simulink model "ModeStEnCtrl6s7sPreCondition"  (R2018b)
settings: Solver=FixedStepDiscrete  StartTime=0.0  StopTime=10.0  RelTol=1e-3
undefined symbols (not defined in the file or in its folder): KeSMSuSecRwStBackPosDelta_Val
libraries: simulink x2
settings Model: Creator=sn2xws  LastModifiedBy=sn2xws
settings DataIOCC: SaveFormat=StructureWithTime
settings OptimizationCC: DefaultParameterBehavior=Inlined  EnhancedBackFolding=on  PassReuseOutputArgsAs=Individual arguments  ZeroExternalMemoryAtStartup=off  ZeroInternalMemoryAtStartup=off  OptimizeBlockOrder=speed  DifferentSizesBufferReuse=on  OptimizationCustomize=off
settings DebuggingCC: ParameterTunabilityLossMsg=error
settings SFSimCC: MATLABDynamicMemAlloc=off
settings RTWCC: SystemTargetFile=autosar.tlc  GenCodeOnly=on  TemplateMakefile=ert_default_tmf  Description=AUTOSAR  GenerateReport=on  IncludeHyperlinkInReport=on  LaunchReport=on  GenerateTraceInfo=on  GenerateTraceReport=on  GenerateTraceReportSl=on  GenerateTraceReportSf=on  GenerateTraceReportEml=on  GenerateCodeMetricsReport=on
settings CodeAppCC: ForceParamTrailComments=on  IgnoreCustomStorageClasses=off  OperatorAnnotations=on  SimulinkDataObjDesc=on  SFDataObjDesc=on  InsertBlockDesc=on
settings STFCustomTargetCC: TargetLangStandard=C99 (ISO)  MultiwordLength=256  ParMdlRefBuildCompliant=on  CompOptLevelCompliant=on  IncludeMdlTerminateFcn=off  CombineOutputUpdateFcns=on  SuppressErrorStatus=on  ERTCustomFileBanners=on  SupportNonFinite=off  SupportComplex=off  SupportContinuousTime=off  SupportNonInlinedSFcns=off  RemoveResetFunc=on  MATLABClassNameForMDSCustomization=Simulink.SoftwareTarget.ERTCustomization  AutosarCompliant=on  UseToolchainInfoCompliant=on  LookupTableObjectStructAxisOrder=2,1,3,4,...  LUTObjectStructOrderEvenSpacing=Size,Table,Breakpoints  SystemTargetFile=autosar.tlc
settings ERTTargetCC: TargetLangStandard=C99 (ISO)  ConcurrentExecutionCompliant=off  IncludeMdlTerminateFcn=off  SuppressErrorStatus=on  SupportNonFinite=off  SupportComplex=off  ModelStepFunctionPrototypeControlCompliant=off  CPPClassGenCompliant=off  AutosarCompliant=on  LookupTableObjectStructAxisOrder=2,1,3,4,...  LUTObjectStructOrderEvenSpacing=Size,Table,Breakpoints  InlinedParameterPlacement=NonHierarchical  ERTCustomFileTemplate=example_file_process.tlc  ERTFilePackagingFormat=Compact

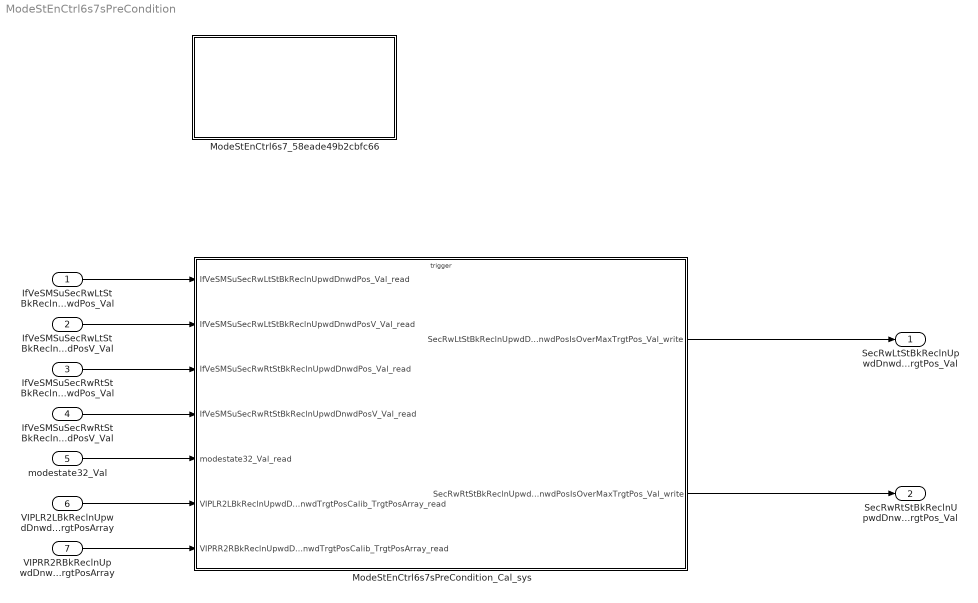
== system ModeStEnCtrl6s7sPreCondition ==
  IfVeSMSuSecRwLtStBkReclnUpwdDnwdPos_Val : Inport  OutDataTypeStr=uint16  PortDimensions=1
  IfVeSMSuSecRwLtStBkReclnUpwdDnwdPosV_Val : Inport  Port=2  OutDataTypeStr=boolean  PortDimensions=1
  IfVeSMSuSecRwRtStBkReclnUpwdDnwdPos_Val : Inport  Port=3  OutDataTypeStr=uint16  PortDimensions=1
  IfVeSMSuSecRwRtStBkReclnUpwdDnwdPosV_Val : Inport  Port=4  OutDataTypeStr=boolean  PortDimensions=1
  modestate32_Val : Inport  Port=5  OutDataTypeStr=uint32  PortDimensions=1
  VIPLR2LBkReclnUpwdDnwdTrgtPosCalib_TrgtPosArray : Inport  Description=|  Port=6  OutDataTypeStr=uint16  PortDimensions=3
      | 0:Pos
      | 1:Max
      | 2:Min
  VIPRR2RBkReclnUpwdDnwdTrgtPosCalib_TrgtPosArray : Inport  Description=|  Port=7  OutDataTypeStr=uint16  PortDimensions=3
      | 0:Pos
      | 1:Max
      | 2:Min
  ModeStEnCtrl6s7_58eade49b2cbfc66 : Subsystem
  ModeStEnCtrl6s7sPreCondition_Cal_sys : Subsystem
  SecRwLtStBkReclnUpwdDnwdPosIsOverMaxTrgtPos_Val : Outport  OutDataTypeStr=boolean  PortDimensions=1
  SecRwRtStBkReclnUpwdDnwdPosIsOverMaxTrgtPos_Val : Outport  Port=2  OutDataTypeStr=boolean  PortDimensions=1
  wires:
  IfVeSMSuSecRwLtStBkReclnUpwdDnwdPos_Val/1 -> ModeStEnCtrl6s7sPreCondition_Cal_sys/1(IfVeSMSuSecRwLtStBkReclnUpwdDnwdPos_Val_read)
  IfVeSMSuSecRwLtStBkReclnUpwdDnwdPosV_Val/1 -> ModeStEnCtrl6s7sPreCondition_Cal_sys/2(IfVeSMSuSecRwLtStBkReclnUpwdDnwdPosV_Val_read)
  IfVeSMSuSecRwRtStBkReclnUpwdDnwdPos_Val/1 -> ModeStEnCtrl6s7sPreCondition_Cal_sys/3(IfVeSMSuSecRwRtStBkReclnUpwdDnwdPos_Val_read)
  IfVeSMSuSecRwRtStBkReclnUpwdDnwdPosV_Val/1 -> ModeStEnCtrl6s7sPreCondition_Cal_sys/4(IfVeSMSuSecRwRtStBkReclnUpwdDnwdPosV_Val_read)
  modestate32_Val/1 -> ModeStEnCtrl6s7sPreCondition_Cal_sys/5(modestate32_Val_read)
  VIPLR2LBkReclnUpwdDnwdTrgtPosCalib_TrgtPosArray/1 -> ModeStEnCtrl6s7sPreCondition_Cal_sys/6(VIPLR2LBkReclnUpwdDnwdTrgtPosCalib_TrgtPosArray_read)
  VIPRR2RBkReclnUpwdDnwdTrgtPosCalib_TrgtPosArray/1 -> ModeStEnCtrl6s7sPreCondition_Cal_sys/7(VIPRR2RBkReclnUpwdDnwdTrgtPosCalib_TrgtPosArray_read)
  ModeStEnCtrl6s7sPreCondition_Cal_sys/1(SecRwLtStBkReclnUpwdDnwdPosIsOverMaxTrgtPos_Val_write) -> SecRwLtStBkReclnUpwdDnwdPosIsOverMaxTrgtPos_Val/1
  ModeStEnCtrl6s7sPreCondition_Cal_sys/2(SecRwRtStBkReclnUpwdDnwdPosIsOverMaxTrgtPos_Val_write) -> SecRwRtStBkReclnUpwdDnwdPosIsOverMaxTrgtPos_Val/1

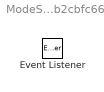
== system ModeStEnCtrl6s7sPreCondition/ModeStEnCtrl6s7_58eade49b2cbfc66 ==
  Event Listener : EventListener  EventName=reset

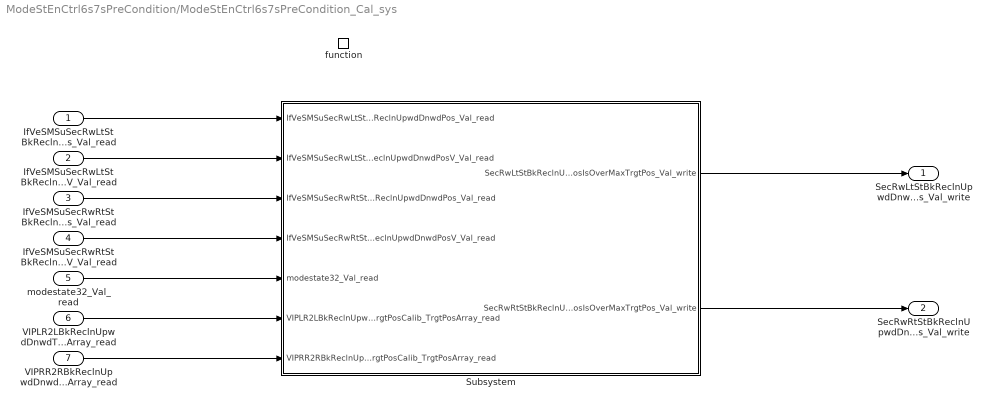
== system ModeStEnCtrl6s7sPreCondition/ModeStEnCtrl6s7sPreCondition_Cal_sys ==
  IfVeSMSuSecRwLtStBkReclnUpwdDnwdPos_Val_read : Inport
  IfVeSMSuSecRwLtStBkReclnUpwdDnwdPosV_Val_read : Inport  Port=2
  IfVeSMSuSecRwRtStBkReclnUpwdDnwdPos_Val_read : Inport  Port=3
  IfVeSMSuSecRwRtStBkReclnUpwdDnwdPosV_Val_read : Inport  Port=4
  modestate32_Val_read : Inport  Port=5
  VIPLR2LBkReclnUpwdDnwdTrgtPosCalib_TrgtPosArray_read : Inport  Port=6
  VIPRR2RBkReclnUpwdDnwdTrgtPosCalib_TrgtPosArray_read : Inport  Port=7
  function : TriggerPort  TriggerType=function-call  IsSimulinkFunction=on  FunctionName=ModeStEnCtrl6s7sPreCondition_Cal  VariantControl=(inherit)
  Subsystem : Subsystem
  SecRwLtStBkReclnUpwdDnwdPosIsOverMaxTrgtPos_Val_write : Outport
      settings: EnsureOutportIsVirtual=on
  SecRwRtStBkReclnUpwdDnwdPosIsOverMaxTrgtPos_Val_write : Outport  Port=2
      settings: EnsureOutportIsVirtual=on
  wires:
  IfVeSMSuSecRwLtStBkReclnUpwdDnwdPos_Val_read/1 -> Subsystem/1(IfVeSMSuSecRwLtStBkReclnUpwdDnwdPos_Val_read)
  IfVeSMSuSecRwLtStBkReclnUpwdDnwdPosV_Val_read/1 -> Subsystem/2(IfVeSMSuSecRwLtStBkReclnUpwdDnwdPosV_Val_read)
  IfVeSMSuSecRwRtStBkReclnUpwdDnwdPos_Val_read/1 -> Subsystem/3(IfVeSMSuSecRwRtStBkReclnUpwdDnwdPos_Val_read)
  IfVeSMSuSecRwRtStBkReclnUpwdDnwdPosV_Val_read/1 -> Subsystem/4(IfVeSMSuSecRwRtStBkReclnUpwdDnwdPosV_Val_read)
  modestate32_Val_read/1 -> Subsystem/5(modestate32_Val_read)
  VIPLR2LBkReclnUpwdDnwdTrgtPosCalib_TrgtPosArray_read/1 -> Subsystem/6(VIPLR2LBkReclnUpwdDnwdTrgtPosCalib_TrgtPosArray_read)
  VIPRR2RBkReclnUpwdDnwdTrgtPosCalib_TrgtPosArray_read/1 -> Subsystem/7(VIPRR2RBkReclnUpwdDnwdTrgtPosCalib_TrgtPosArray_read)
  Subsystem/1(SecRwLtStBkReclnUpwdDnwdPosIsOverMaxTrgtPos_Val_write) -> SecRwLtStBkReclnUpwdDnwdPosIsOverMaxTrgtPos_Val_write/1
  Subsystem/2(SecRwRtStBkReclnUpwdDnwdPosIsOverMaxTrgtPos_Val_write) -> SecRwRtStBkReclnUpwdDnwdPosIsOverMaxTrgtPos_Val_write/1

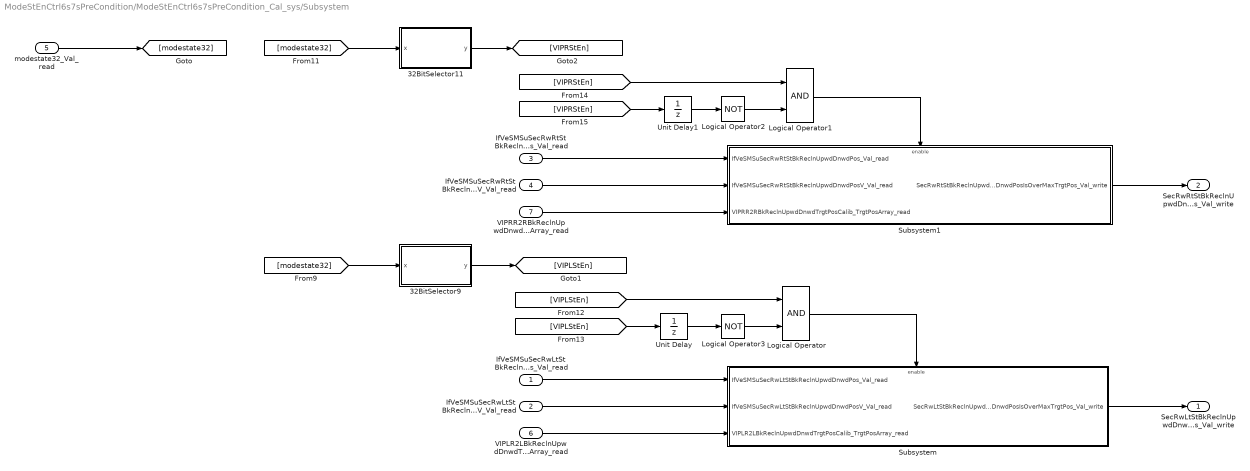
== system ModeStEnCtrl6s7sPreCondition/ModeStEnCtrl6s7sPreCondition_Cal_sys/Subsystem ==
  IfVeSMSuSecRwLtStBkReclnUpwdDnwdPos_Val_read : Inport
  IfVeSMSuSecRwLtStBkReclnUpwdDnwdPosV_Val_read : Inport  Port=2
  IfVeSMSuSecRwRtStBkReclnUpwdDnwdPos_Val_read : Inport  Port=3
  IfVeSMSuSecRwRtStBkReclnUpwdDnwdPosV_Val_read : Inport  Port=4
  modestate32_Val_read : Inport  Port=5
  VIPLR2LBkReclnUpwdDnwdTrgtPosCalib_TrgtPosArray_read : Inport  Port=6
  VIPRR2RBkReclnUpwdDnwdTrgtPosCalib_TrgtPosArray_read : Inport  Port=7
  32BitSelector11 : Subsystem  mask(32 Bit Selector){BitNum=11}
      mask prompts: BitNum "Select Bit Number"
      mask help: Allows selection of a particular bit (0-31) out of a packed word up to 32 bits long. Output will be true if the bit number selected via the mask parameter is equal to one.
      mask TypeOptions BitNum: 0 | 1 | 2 | 3 | 4 | 5 | 6 | 7 | 8 | 9 | 10 | 11 | 12 | 13 | 14 | 15 | 16 | 17 | 18 | 19 | 20 | 21 | 22 | 23 | 24 | 25 | 26 | 27 | 28 | 29 | 30 | 31
      mask Display:
      | text(0.5, 0.8,'BIT','horizontalAlignment','center')
      | text(0.5, 0.5,'SELECTOR','horizontalAlignment','center')
      | text(0.5, 0.2,['-- Bit ',char(get_param(gcb,'BitNum')),' --'],'horizontalAlignment','center')
  32BitSelector9 : Subsystem  mask(32 Bit Selector){BitNum=9}
      mask prompts: BitNum "Select Bit Number"
      mask help: Allows selection of a particular bit (0-31) out of a packed word up to 32 bits long. Output will be true if the bit number selected via the mask parameter is equal to one.
      mask TypeOptions BitNum: 0 | 1 | 2 | 3 | 4 | 5 | 6 | 7 | 8 | 9 | 10 | 11 | 12 | 13 | 14 | 15 | 16 | 17 | 18 | 19 | 20 | 21 | 22 | 23 | 24 | 25 | 26 | 27 | 28 | 29 | 30 | 31
      mask Display:
      | text(0.5, 0.8,'BIT','horizontalAlignment','center')
      | text(0.5, 0.5,'SELECTOR','horizontalAlignment','center')
      | text(0.5, 0.2,['-- Bit ',char(get_param(gcb,'BitNum')),' --'],'horizontalAlignment','center')
  Logical Operator : Logic  AllPortsSameDT=off  OutDataTypeStr=boolean
  Logical Operator1 : Logic  AllPortsSameDT=off  OutDataTypeStr=boolean
  Logical Operator2 : Logic  Operator=NOT  AllPortsSameDT=off  OutDataTypeStr=boolean
  Logical Operator3 : Logic  Operator=NOT  AllPortsSameDT=off  OutDataTypeStr=boolean
  Subsystem : Subsystem
  Subsystem1 : Subsystem
  Unit Delay : UnitDelay  SampleTime=-1
  Unit Delay1 : UnitDelay  SampleTime=-1
  SecRwLtStBkReclnUpwdDnwdPosIsOverMaxTrgtPos_Val_write : Outport
      settings: EnsureOutportIsVirtual=on
  SecRwRtStBkReclnUpwdDnwdPosIsOverMaxTrgtPos_Val_write : Outport  Port=2
      settings: EnsureOutportIsVirtual=on
  wires:
  IfVeSMSuSecRwRtStBkReclnUpwdDnwdPos_Val_read/1 -> Subsystem1/1(IfVeSMSuSecRwRtStBkReclnUpwdDnwdPos_Val_read)
  IfVeSMSuSecRwLtStBkReclnUpwdDnwdPosV_Val_read/1 -> Subsystem/2(IfVeSMSuSecRwLtStBkReclnUpwdDnwdPosV_Val_read)
  IfVeSMSuSecRwLtStBkReclnUpwdDnwdPos_Val_read/1 -> Subsystem/1(IfVeSMSuSecRwLtStBkReclnUpwdDnwdPos_Val_read)
  IfVeSMSuSecRwRtStBkReclnUpwdDnwdPosV_Val_read/1 -> Subsystem1/2(IfVeSMSuSecRwRtStBkReclnUpwdDnwdPosV_Val_read)
  VIPLR2LBkReclnUpwdDnwdTrgtPosCalib_TrgtPosArray_read/1 -> Subsystem/3(VIPLR2LBkReclnUpwdDnwdTrgtPosCalib_TrgtPosArray_read)
  [modestate32] -> 32BitSelector11/1(x)
  32BitSelector11/1(y) -> [VIPRStEn]
  modestate32_Val_read/1 -> [modestate32]
  [VIPRStEn] -> Unit Delay1/1
  Logical Operator1/1 -> Subsystem1/Enable
  Unit Delay1/1 -> Logical Operator2/1
  [VIPRStEn] -> Logical Operator1/1
  VIPRR2RBkReclnUpwdDnwdTrgtPosCalib_TrgtPosArray_read/1 -> Subsystem1/3(VIPRR2RBkReclnUpwdDnwdTrgtPosCalib_TrgtPosArray_read)
  Subsystem1/1(SecRwRtStBkReclnUpwdDnwdPosIsOverMaxTrgtPos_Val_write) -> SecRwRtStBkReclnUpwdDnwdPosIsOverMaxTrgtPos_Val_write/1
  Subsystem/1(SecRwLtStBkReclnUpwdDnwdPosIsOverMaxTrgtPos_Val_write) -> SecRwLtStBkReclnUpwdDnwdPosIsOverMaxTrgtPos_Val_write/1
  Logical Operator/1 -> Subsystem/Enable
  [VIPLStEn] -> Unit Delay/1
  [VIPLStEn] -> Logical Operator/1
  Unit Delay/1 -> Logical Operator3/1
  32BitSelector9/1(y) -> [VIPLStEn]
  [modestate32] -> 32BitSelector9/1(x)
  Logical Operator2/1 -> Logical Operator1/2
  Logical Operator3/1 -> Logical Operator/2

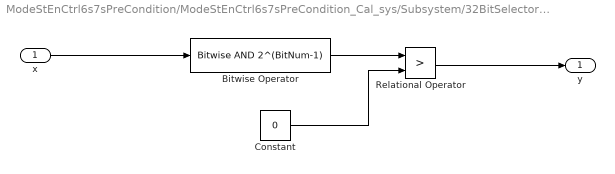
== system ModeStEnCtrl6s7sPreCondition/ModeStEnCtrl6s7sPreCondition_Cal_sys/Subsystem/32BitSelector11 ==
  x : Inport
  Bitwise Operator : simulink/Logic and Bit Operations/Bitwise Operator  logicop=AND  UseBitMask=on  BitMask=2^(BitNum-1)  BitMaskRealWorld=Stored Integer
  Constant : Constant  Value=0  OutDataTypeStr=uint32
  Relational Operator : RelationalOperator  Operator=>  OutDataTypeStr=boolean  RndMeth=Simplest
  y : Outport
  wires:
  Bitwise Operator/1 -> Relational Operator/1
  x/1 -> Bitwise Operator/1
  Constant/1 -> Relational Operator/2
  Relational Operator/1 -> y/1

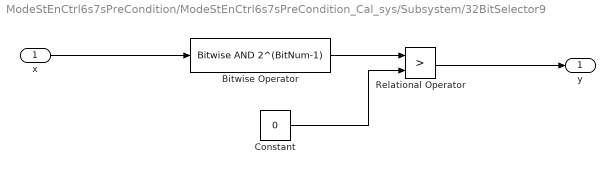
== system ModeStEnCtrl6s7sPreCondition/ModeStEnCtrl6s7sPreCondition_Cal_sys/Subsystem/32BitSelector9 ==
  x : Inport
  Bitwise Operator : simulink/Logic and Bit Operations/Bitwise Operator  logicop=AND  UseBitMask=on  BitMask=2^(BitNum-1)  BitMaskRealWorld=Stored Integer
  Constant : Constant  Value=0  OutDataTypeStr=uint32
  Relational Operator : RelationalOperator  Operator=>  OutDataTypeStr=boolean  RndMeth=Simplest
  y : Outport
  wires:
  Bitwise Operator/1 -> Relational Operator/1
  x/1 -> Bitwise Operator/1
  Constant/1 -> Relational Operator/2
  Relational Operator/1 -> y/1

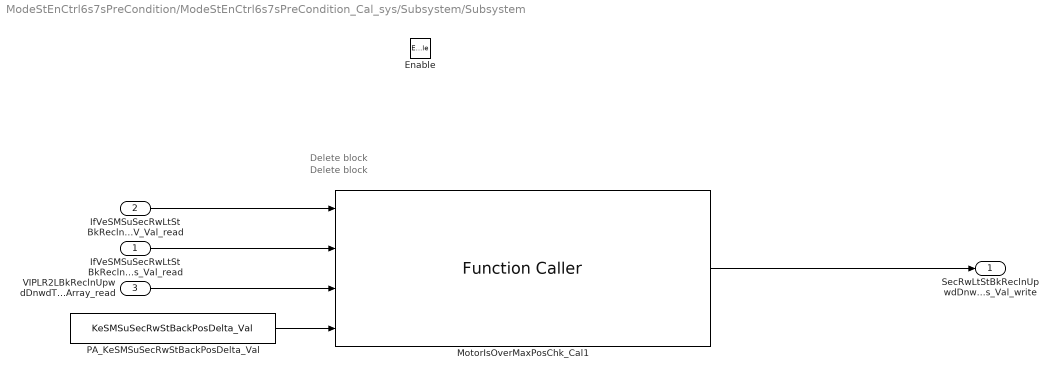
== system ModeStEnCtrl6s7sPreCondition/ModeStEnCtrl6s7sPreCondition_Cal_sys/Subsystem/Subsystem ==
  note: Delete block
  note: Delete block
  IfVeSMSuSecRwLtStBkReclnUpwdDnwdPos_Val_read : Inport
  IfVeSMSuSecRwLtStBkReclnUpwdDnwdPosV_Val_read : Inport  Port=2
  VIPLR2LBkReclnUpwdDnwdTrgtPosCalib_TrgtPosArray_read : Inport  Port=3
  Enable : EnablePort
  MotorIsOverMaxPosChk_Cal1 : FunctionCaller  FunctionPrototype=IsOverMaxTrgtPos = MotorIsOverMaxPosChk_Cal(PosV,Pos,TrgtPosCalib,Delta)  InputArgumentSpecifications=boolean(true), uint16(1), uint16([1;1;1]), uint16(1)  OutputArgumentSpecifications=boolean(true)
  PA_KeSMSuSecRwStBackPosDelta_Val : Constant  Value=KeSMSuSecRwStBackPosDelta_Val
  SecRwLtStBkReclnUpwdDnwdPosIsOverMaxTrgtPos_Val_write : Outport
      settings: EnsureOutportIsVirtual=on
  wires:
  PA_KeSMSuSecRwStBackPosDelta_Val/1 -> MotorIsOverMaxPosChk_Cal1/4
  VIPLR2LBkReclnUpwdDnwdTrgtPosCalib_TrgtPosArray_read/1 -> MotorIsOverMaxPosChk_Cal1/3
  IfVeSMSuSecRwLtStBkReclnUpwdDnwdPos_Val_read/1 -> MotorIsOverMaxPosChk_Cal1/2
  IfVeSMSuSecRwLtStBkReclnUpwdDnwdPosV_Val_read/1 -> MotorIsOverMaxPosChk_Cal1/1
  MotorIsOverMaxPosChk_Cal1/1 -> SecRwLtStBkReclnUpwdDnwdPosIsOverMaxTrgtPos_Val_write/1

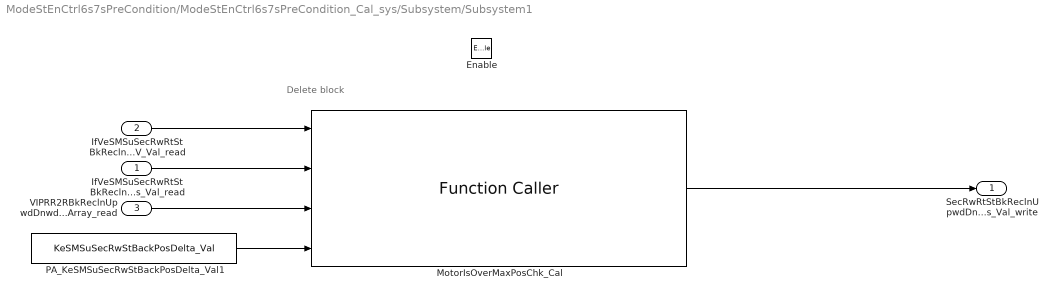
== system ModeStEnCtrl6s7sPreCondition/ModeStEnCtrl6s7sPreCondition_Cal_sys/Subsystem/Subsystem1 ==
  note: Delete block
  IfVeSMSuSecRwRtStBkReclnUpwdDnwdPos_Val_read : Inport
  IfVeSMSuSecRwRtStBkReclnUpwdDnwdPosV_Val_read : Inport  Port=2
  VIPRR2RBkReclnUpwdDnwdTrgtPosCalib_TrgtPosArray_read : Inport  Port=3
  Enable : EnablePort
  MotorIsOverMaxPosChk_Cal : FunctionCaller  FunctionPrototype=IsOverMaxTrgtPos = MotorIsOverMaxPosChk_Cal(PosV,Pos,TrgtPosCalib,Delta)  InputArgumentSpecifications=boolean(true), uint16(1), uint16([1;1;1]), uint16(1)  OutputArgumentSpecifications=boolean(true)
  PA_KeSMSuSecRwStBackPosDelta_Val1 : Constant  Value=KeSMSuSecRwStBackPosDelta_Val
  SecRwRtStBkReclnUpwdDnwdPosIsOverMaxTrgtPos_Val_write : Outport
      settings: EnsureOutportIsVirtual=on
  wires:
  VIPRR2RBkReclnUpwdDnwdTrgtPosCalib_TrgtPosArray_read/1 -> MotorIsOverMaxPosChk_Cal/3
  PA_KeSMSuSecRwStBackPosDelta_Val1/1 -> MotorIsOverMaxPosChk_Cal/4
  IfVeSMSuSecRwRtStBkReclnUpwdDnwdPos_Val_read/1 -> MotorIsOverMaxPosChk_Cal/2
  MotorIsOverMaxPosChk_Cal/1 -> SecRwRtStBkReclnUpwdDnwdPosIsOverMaxTrgtPos_Val_write/1
  IfVeSMSuSecRwRtStBkReclnUpwdDnwdPosV_Val_read/1 -> MotorIsOverMaxPosChk_Cal/1
